simulink model "W3P3"  (R2020b)
settings: Solver=VariableStepAuto  StartTime=0.0  StopTime=10.0  RelTol=1e-3
values from neighbouring files (symbols this model uses):
  g = 9.01    [DATA.sldd]    (also in matlab.mat = 9.81)
  I = 6.0    [DATA.sldd]    (also in matlab.mat = 6)
  m = 75.0    [DATA.sldd]    (also in matlab.mat = 75)
  R = 1.25    [DATA.sldd]    (also in matlab.mat)
  v0 = 44.0    [DATA.sldd]    (also in matlab.mat = 44)
settings Model: Creator=ASUS  LastModifiedBy=ASUS

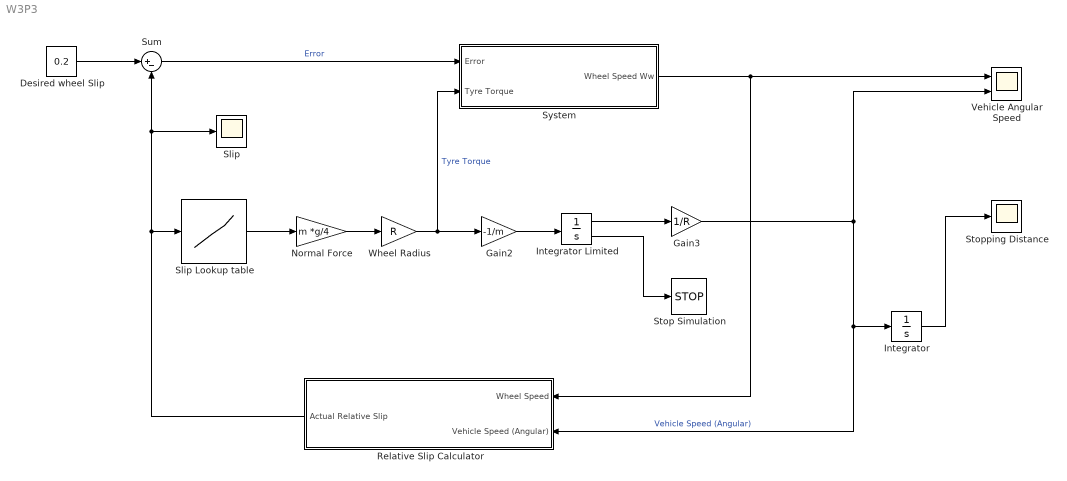
== system W3P3 ==
  Desired wheel Slip : Constant  Value=0.2
  Gain2 : Gain  Gain=-1/m
  Gain3 : Gain  Gain=1/R
  Integrator : Integrator
  Integrator Limited : Integrator  InitialCondition=v0  LimitOutput=on  UpperSaturationLimit=1000  LowerSaturationLimit=0  ShowSaturationPort=on
  Normal Force : Gain  Gain=m *g/4
  Relative Slip Calculator : Subsystem
  Slip : Scope
  Slip Lookup table : Lookup_n-D  NumberOfTableDimensions=1  BreakpointsForDimension1=[0,0.05,0.1,0.15,0.2,0.25,0.3,0.35,0.4,0.45,0.5,0.55,0.6,0.65,0.7,0.75,0.8,0.85,0.9,0.95,1]  Table=[0,0.4,0.8,0.97,1,0.98,0.96,0.94,0.92,0.9,0.88,0.855,0.83,0.81,0.79,0.77,0.75,0.73,0.72,0.71,0.7]  InternalRulePriority=Speed  RndMeth=Simplest  InputSameDT=on
  Stop Simulation : Stop
  Stopping Distance : Scope
  Sum : Sum  Inputs=|+-
  System : Subsystem
  "Vehicle Angular Speed " : Scope  NumInputPorts=2
  Wheel Radius : Gain  Gain=R
  wires:
  Desired wheel Slip/1 -> Sum/1
  Slip Lookup table/1 -> Normal Force/1
  Normal Force/1 -> Wheel Radius/1
  Sum/1 -> System/1(Error)  "Error"
  Wheel Radius/1 -> Gain2/1, System/2(Tyre Torque)  "Tyre Torque"
  System/1(Wheel Speed Ww) -> "Vehicle Angular Speed "/1, Relative Slip Calculator/1(Wheel Speed)
  Gain2/1 -> Integrator Limited/1
  Integrator Limited/1 -> Gain3/1
  Gain3/1 -> "Vehicle Angular Speed "/2, Integrator/1, Relative Slip Calculator/2(Vehicle Speed (Angular))  "Vehicle Speed (Angular)"
  Integrator Limited/2 -> Stop Simulation/1
  Integrator/1 -> Stopping Distance/1
  Relative Slip Calculator/1(Actual Relative Slip) -> Slip/1, Sum/2, Slip Lookup table/1

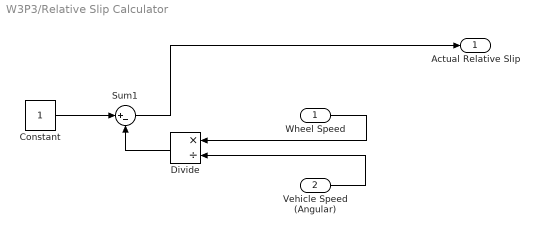
== system W3P3/Relative Slip Calculator ==
  Wheel Speed : Inport
  Vehicle Speed (Angular) : Inport  Port=2
  Constant : Constant
  Divide : Product  Inputs=*/
  Sum1 : Sum  Inputs=|+-
  Actual Relative Slip : Outport
  wires:
  Divide/1 -> Sum1/2
  Constant/1 -> Sum1/1
  Wheel Speed/1 -> Divide/1
  Vehicle Speed (Angular)/1 -> Divide/2
  Sum1/1 -> Actual Relative Slip/1

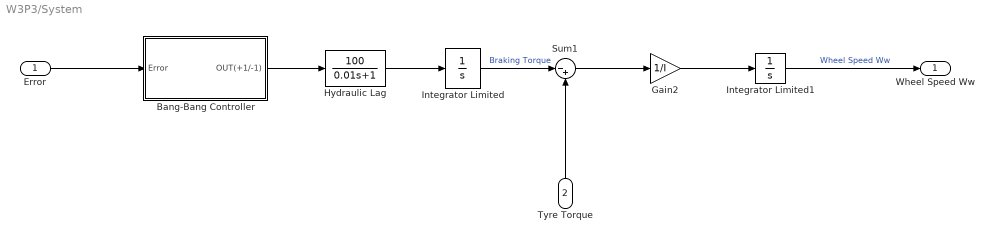
== system W3P3/System ==
  Error : Inport
  Tyre Torque : Inport  Port=2
  Bang-Bang Controller : Subsystem
  Gain2 : Gain  Gain=1/I
  Hydraulic Lag : TransferFcn  Numerator=[100]  Denominator=[0.01 1]
  Integrator Limited : Integrator  LimitOutput=on  UpperSaturationLimit=1000  LowerSaturationLimit=0
  Integrator Limited1 : Integrator  InitialCondition=v0/R  LimitOutput=on  UpperSaturationLimit=1000  LowerSaturationLimit=0
  Sum1 : Sum  Inputs=|-+
  Wheel Speed Ww : Outport
  wires:
  Sum1/1 -> Gain2/1
  Gain2/1 -> Integrator Limited1/1
  Integrator Limited/1 -> Sum1/1  "Braking Torque"
  Bang-Bang Controller/1(OUT(+1/-1)) -> Hydraulic Lag/1
  Error/1 -> Bang-Bang Controller/1(Error)
  Hydraulic Lag/1 -> Integrator Limited/1
  Tyre Torque/1 -> Sum1/2
  Integrator Limited1/1 -> Wheel Speed Ww/1  "Wheel Speed Ww"

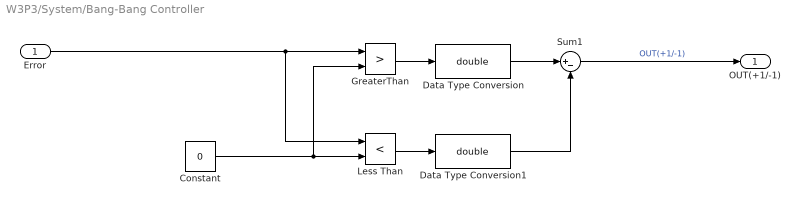
== system W3P3/System/Bang-Bang Controller ==
  Error : Inport
  Constant : Constant  Value=0
  Data Type Conversion : DataTypeConversion  OutDataTypeStr=double  RndMeth=Zero
  Data Type Conversion1 : DataTypeConversion  OutDataTypeStr=double  RndMeth=Zero
  GreaterThan : RelationalOperator  Operator=>  OutDataTypeStr=boolean  RndMeth=Simplest
  Less Than : RelationalOperator  Operator=<  OutDataTypeStr=boolean  RndMeth=Simplest
  Sum1 : Sum  Inputs=|+-
  OUT(+1/-1) : Outport
  wires:
  Data Type Conversion/1 -> Sum1/1
  Constant/1 -> Less Than/2, GreaterThan/2
  Less Than/1 -> Data Type Conversion1/1
  GreaterThan/1 -> Data Type Conversion/1
  Error/1 -> GreaterThan/1, Less Than/1
  Data Type Conversion1/1 -> Sum1/2
  Sum1/1 -> OUT(+1/-1)/1  "OUT(+1/-1)"
